simulink model "MRAC_Lab2"  (R2020a)
settings: Solver=VariableStepAuto  StartTime=0.0  StopTime=50  RelTol=1e-3
model workspace (MAT data in the model file):
  gamma = Simulink.Parameter
  gamma.Value = 0.01
  gamma.DataType = 'auto'
  gamma.Dimensions = [1 1]
undefined symbols (not defined in the file): den, num
settings Model: Creator=Lenovo  LastModifiedBy=Lenovo

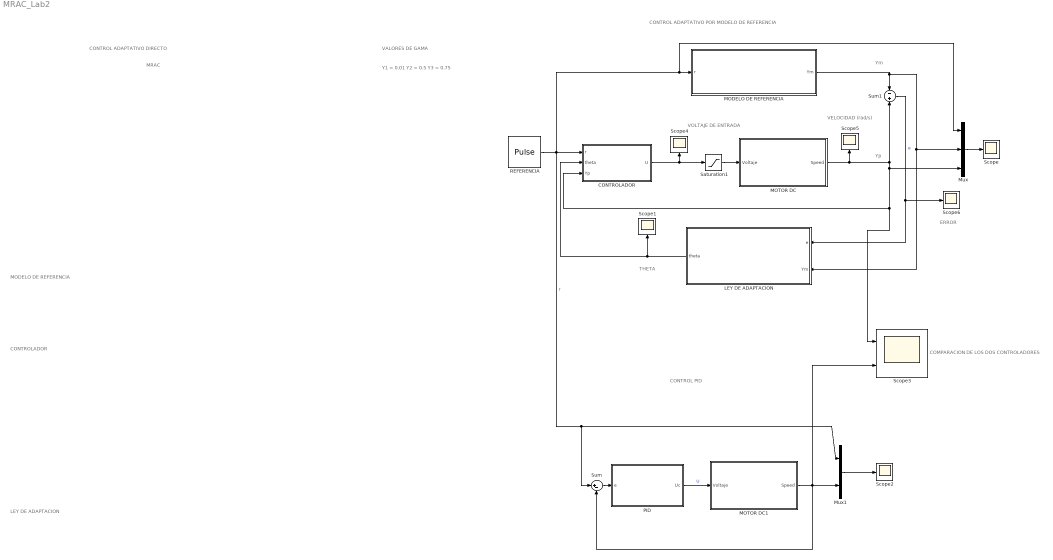
== system MRAC_Lab2 ==
  note: ERROR
  note: COMPARACION DE LOS DOS CONTROLADORES
  note: CONTROL PID
  note: CONTROL ADAPTATIVO POR MODELO DE REFERENCIA
  note: VELOCIDAD (rad/s)
  note: THETA
  note: VOLTAJE DE ENTRADA
  note: LEY DE ADAPTACION
  note: CONTROLADOR
  note: MODELO DE REFERENCIA
  note: MRAC
  note: CONTROL ADAPTATIVO DIRECTO
  note: Y1 = 0.01
      | Y2 = 0.5
      | Y3 = 0.75
  note: VALORES DE GAMA
  note: Ym
  note: Yp
  CONTROLADOR : Subsystem
  LEY DE ADAPTACION : Subsystem
  MODELO DE REFERENCIA : Subsystem
  MOTOR DC : Subsystem
  MOTOR DC1 : Subsystem
  Mux : Mux  Inputs=3
  Mux1 : Mux  Inputs=2
  PID : Subsystem
  REFERENCIA : DiscretePulseGenerator  PulseType=Time based  Amplitude=300  Period=10  PulseWidth=50
  Saturation1 : Saturate  UpperLimit=18  LowerLimit=0
  Scope{,1..2,4..6} (6 alike) : Scope
  Scope3 : Scope  NumInputPorts=2
  Sum : Sum  Inputs=|+-
  Sum1 : Sum  Inputs=-|+
  wires:
  MODELO DE REFERENCIA/1(Ym) -> Sum1/1, LEY DE ADAPTACION/2(Ym), Mux/2
  CONTROLADOR/1(U) -> Saturation1/1, Scope4/1
  MOTOR DC/1(Speed) -> Mux/3, Scope3/1, CONTROLADOR/3(Yp), Sum1/2, Scope5/1
  Sum1/1 -> Scope6/1, LEY DE ADAPTACION/1(e)  "e"
  Mux/1 -> Scope/1
  LEY DE ADAPTACION/1(theta) -> CONTROLADOR/2(theta), Scope1/1
  REFERENCIA/1 -> CONTROLADOR/1(r), Sum/1, Mux1/1, Mux/1, MODELO DE REFERENCIA/1(r)  "r"
  MOTOR DC1/1(Speed) -> Scope3/2, Sum/2, Mux1/2
  Sum/1 -> PID/1(e)
  PID/1(Uc) -> MOTOR DC1/1(Voltaje)  "U"
  Mux1/1 -> Scope2/1
  Saturation1/1 -> MOTOR DC/1(Voltaje)

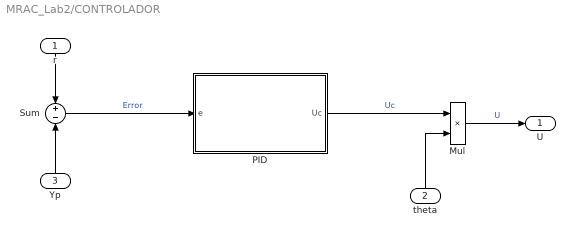
== system MRAC_Lab2/CONTROLADOR ==
  r : Inport
  theta : Inport  Port=2
  Yp : Inport  Port=3
  Mul : Product
  PID : Subsystem
  Sum : Sum  Inputs=+|-
  U : Outport  VectorParamsAs1DForOutWhenUnconnected=off
  wires:
  theta/1 -> Mul/2
  r/1 -> Sum/1
  Yp/1 -> Sum/2
  PID/1(Uc) -> Mul/1  "Uc"
  Sum/1 -> PID/1(e)  "Error"
  Mul/1 -> U/1  "U"

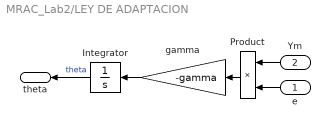
== system MRAC_Lab2/LEY DE ADAPTACION ==
  e : Inport
  Ym : Inport  Port=2
  Integrator : Integrator  InitialCondition=1
  Product : Product
  gamma : Gain  Gain=-gamma
  theta : Outport  VectorParamsAs1DForOutWhenUnconnected=off
  wires:
  Integrator/1 -> theta/1  "theta"
  gamma/1 -> Integrator/1
  Product/1 -> gamma/1
  Ym/1 -> Product/1
  e/1 -> Product/2

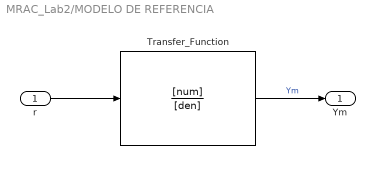
== system MRAC_Lab2/MODELO DE REFERENCIA ==
  r : Inport
  Transfer_Function : TransferFcn  Numerator=[num]  Denominator=[den]
  Ym : Outport  VectorParamsAs1DForOutWhenUnconnected=off
  wires:
  Transfer_Function/1 -> Ym/1  "Ym"
  r/1 -> Transfer_Function/1

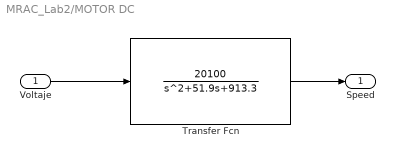
== system MRAC_Lab2/MOTOR DC ==
  Voltaje : Inport
  Transfer Fcn : TransferFcn  Numerator=[20100]  Denominator="[1   51.9  913.3]"
  Speed : Outport
  wires:
  Transfer Fcn/1 -> Speed/1
  Voltaje/1 -> Transfer Fcn/1

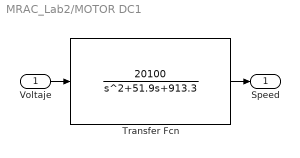
== system MRAC_Lab2/MOTOR DC1 ==
  Voltaje : Inport
  Transfer Fcn : TransferFcn  Numerator=[20100]  Denominator="[1   51.9  913.3]"
  Speed : Outport
  wires:
  Transfer Fcn/1 -> Speed/1
  Voltaje/1 -> Transfer Fcn/1

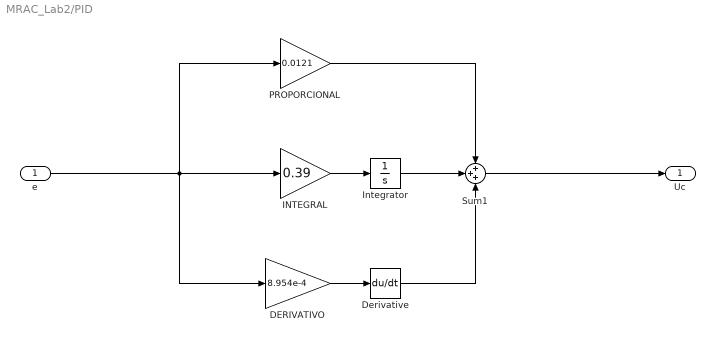
== system MRAC_Lab2/PID ==
  e : Inport
  DERIVATIVO : Gain  Gain=8.954e-4
  Derivative : Derivative
  INTEGRAL : Gain  Gain=0.39
  Integrator : Integrator
  PROPORCIONAL : Gain  Gain=0.0121
  Sum1 : Sum  Inputs=+++
  Uc : Outport
  wires:
  Sum1/1 -> Uc/1
  INTEGRAL/1 -> Integrator/1
  Integrator/1 -> Sum1/2
  e/1 -> DERIVATIVO/1, INTEGRAL/1, PROPORCIONAL/1
  DERIVATIVO/1 -> Derivative/1
  PROPORCIONAL/1 -> Sum1/1
  Derivative/1 -> Sum1/3

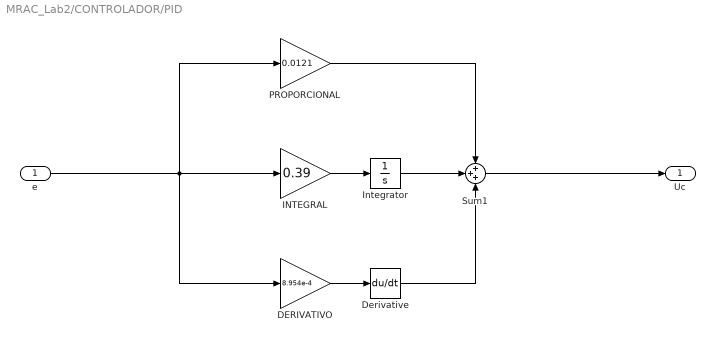
== system MRAC_Lab2/CONTROLADOR/PID ==
  e : Inport
  DERIVATIVO : Gain  Gain=8.954e-4
  Derivative : Derivative
  INTEGRAL : Gain  Gain=0.39
  Integrator : Integrator
  PROPORCIONAL : Gain  Gain=0.0121
  Sum1 : Sum  Inputs=+++
  Uc : Outport
  wires:
  Sum1/1 -> Uc/1
  INTEGRAL/1 -> Integrator/1
  Integrator/1 -> Sum1/2
  e/1 -> DERIVATIVO/1, INTEGRAL/1, PROPORCIONAL/1
  DERIVATIVO/1 -> Derivative/1
  PROPORCIONAL/1 -> Sum1/1
  Derivative/1 -> Sum1/3
